simulink model "sistema_LTI_dinamica_residual"  (R2020b)
settings: Solver=VariableStepAuto  StartTime=0.0  StopTime=1.2  RelTol=1e-3
PreLoadFcn:
  | c4ModeloCompleto_var
PostLoadFcn:
  | c4ModeloCompleto_var
values from neighbouring files (symbols this model uses):
  Beq = bm+(bl)/r^2    (= 1.5e-05)    [c4ModeloCompleto_var.m]
  Jeq = Jm+(Jl/r^2)    (= 5.65099476805e-06)    [c4ModeloCompleto_var.m]
  lambda_m = 0.01546    [c4ModeloCompleto_var.m]
  Ld = 6.6e-3    (= 0.0066)    [c4ModeloCompleto_var.m]
  Lq = 5.8e-3    (= 0.0058)    [c4ModeloCompleto_var.m]
  Pp = 3    [c4ModeloCompleto_var.m]
  r = 314.3008    [c4ModeloCompleto_var.m]
undefined symbols (not defined in the file or in its folder): Rs, sigbuilder_block
settings Model: Creator=agustin  LastModifiedBy=agustin
settings DataIOCC: ReturnWorkspaceOutputs=off
settings DebuggingCC: ArithmeticOperatorsInVariantConditions=warning
settings SFSimCC: SimUseLocalCustomCode=off  CustomCodeUndefinedFunction=UseInterfaceOnly
settings RTWCC: RTWUseLocalCustomCode=off
settings CodeAppCC: StateflowObjectComments=on

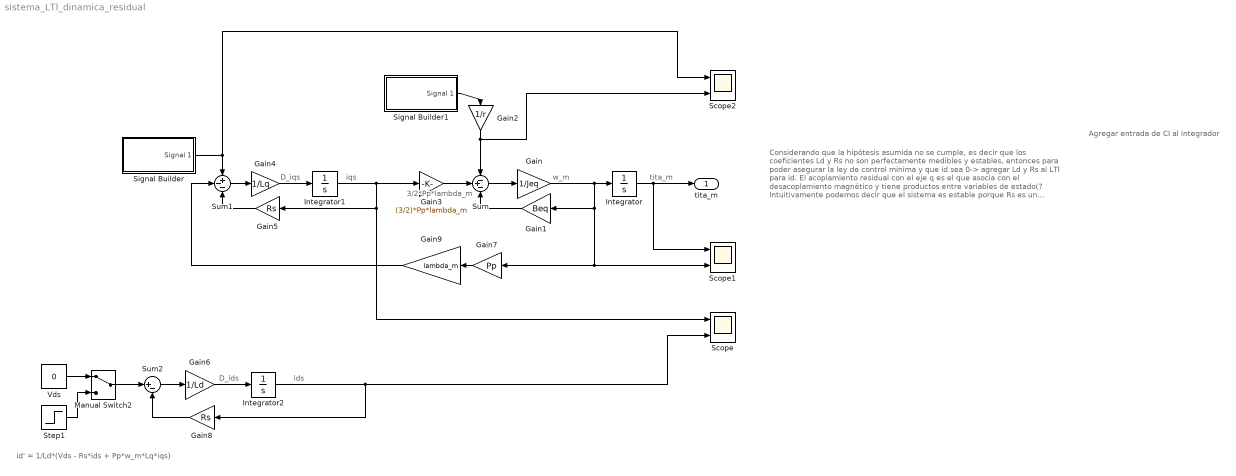
== system sistema_LTI_dinamica_residual ==
  note: id' = 1/Ld*(Vds - Rs*ids + Pp*w_m*Lq*iqs)
  note: 3/2*Pp*lambda_m
  note: Agregar entrada de CI al integrador
  note: Considerando que la hipótesis asumida no se cumple, es decir que los coeficientes Ld y Rs no son perfectamente medibles y estables, entonces para poder asegurar la ley de control mínima y que id sea 0-> agregar Ld y Rs al LTI para id.
      | El acoplamiento residual con el eje q es el que asocia con el desacoplamiento magnético y tiene productos entre variables de estado(?
      |
      | Intuitivamente podemos decir que el sistema es estable porque Rs es un término disipativo, este análisis se ve más en detalle al analizar polos.
      |
      | Se puede llegar a despreciar el acoplamiento NL porque el sistema es estable y se comporta como un filtro pasabajo con una constante de decaimiento Tau (Ld/Rs) que hace converger a la corriente a 0. El comportamiento como pasabajo se debe a que el sistema tiene un polo de primer orden
  note: tita_m
  note: w_m
  note: iqs
  note: D_iqs
  note: ids
  note: D_ids
  Gain : Gain  Gain=1/Jeq
  Gain1 : Gain  Gain=Beq
  Gain2 : Gain  Gain=1/r
  Gain3 : Gain  Gain=(3/2)*Pp*lambda_m
  Gain4 : Gain  Gain=1/Lq
  Gain5 : Gain  Gain=Rs
  Gain6 : Gain  Gain=1/Ld
  Gain7 : Gain  Gain=Pp
  Gain8 : Gain  Gain=Rs
  Gain9 : Gain  Gain=lambda_m
  Integrator : Integrator
  Integrator1 : Integrator
  Integrator2 : Integrator  InitialCondition=-.5
  Manual Switch2 : ManualSwitch
  Scope : Scope  NumInputPorts=2
  Scope1 : Scope  NumInputPorts=2
  Scope2 : Scope  NumInputPorts=2
  Signal Builder : Subsystem  Tag=STV Subsys  LoadFcn=sigbuilder_block('load');  StartFcn=sigbuilder_block('start');  StopFcn=sigbuilder_block('stop');  ClipboardFcn=sigbuilder_block('clipboard');  mask(Sigbuilder block){tuvar=[0:10]}
      mask help: Simulink:masks:SigbuilderBlock_MD
      mask init:
      | if ~strcmp(get_param(bdroot(gcbh),'SimulationStatus'),'stopped') tuvar = sigbuilder_block('maskInit'); end
      settings: CopyFcn=sigbuilder_block('copy');  DeleteFcn=sigbuilder_block('delete');  ModelCloseFcn=sigbuilder_block('modelClose');  PreSaveFcn=sigbuilder_block('preSave');  PauseFcn=sigbuilder_block('pause');  ContinueFcn=sigbuilder_block('continue');  NameChangeFcn=sigbuilder_block('namechange');  OpenFcn=sigbuilder_block('open',[437.25 154.5 550.5 357 ]);  CloseFcn=sigbuilder_block('close');
      mask Display: plot(0, 0, 100, 100,[2, 2, 32, 32, 2], [68, 8, 8, 68, 68],[32, 2], [38, 38], [32, 19, 2],[53, 60, 44], [32, 17, 17, 2],[16, 16, 31, 31]);txt = getActiveGroup(gcbh);text(2, 100, txt,'verticalAlignment', 'top');
  Signal Builder1 : Subsystem  Tag=STV Subsys  LoadFcn=sigbuilder_block('load');  StartFcn=sigbuilder_block('start');  StopFcn=sigbuilder_block('stop');  ClipboardFcn=sigbuilder_block('clipboard');  mask(Sigbuilder block){tuvar=[0:10]}
      mask help: Simulink:masks:SigbuilderBlock_MD
      mask init:
      | if ~strcmp(get_param(bdroot(gcbh),'SimulationStatus'),'stopped') tuvar = sigbuilder_block('maskInit'); end
      settings: CopyFcn=sigbuilder_block('copy');  DeleteFcn=sigbuilder_block('delete');  ModelCloseFcn=sigbuilder_block('modelClose');  PreSaveFcn=sigbuilder_block('preSave');  PauseFcn=sigbuilder_block('pause');  ContinueFcn=sigbuilder_block('continue');  NameChangeFcn=sigbuilder_block('namechange');  OpenFcn=sigbuilder_block('open',[0 0 1024.5 511.5 ]);  CloseFcn=sigbuilder_block('close');
      mask Display: plot(0, 0, 100, 100,[2, 2, 32, 32, 2], [68, 8, 8, 68, 68],[32, 2], [38, 38], [32, 19, 2],[53, 60, 44], [32, 17, 17, 2],[16, 16, 31, 31]);txt = getActiveGroup(gcbh);text(2, 100, txt,'verticalAlignment', 'top');
  Step1 : Step  SampleTime=0
  Sum : Sum  Inputs=-+-
  Sum1 : Sum  Inputs=+--
  Sum2 : Sum  Inputs=|+-
  "Vds " : Constant  Value=0
  tita_m : Outport  VectorParamsAs1DForOutWhenUnconnected=off
  wires:
  Sum/1 -> Gain/1
  Gain1/1 -> Sum/3
  Gain2/1 -> Sum/1, Scope2/2
  Gain3/1 -> Sum/2
  Gain4/1 -> Integrator1/1
  Sum1/1 -> Gain4/1
  Integrator1/1 -> Gain3/1, Gain5/1, Scope/1
  Gain5/1 -> Sum1/3
  Integrator/1 -> Scope1/1, tita_m/1
  Gain/1 -> Scope1/2, Gain7/1, Gain1/1, Integrator/1
  Gain6/1 -> Integrator2/1
  Sum2/1 -> Gain6/1
  Gain8/1 -> Sum2/2
  Gain9/1 -> Sum1/2
  Signal Builder/1(Signal 1) -> Scope2/1, Sum1/1
  Gain7/1 -> Gain9/1
  Signal Builder1/1(Signal 1) -> Gain2/1
  "Vds "/1 -> Manual Switch2/1
  Step1/1 -> Manual Switch2/2
  Manual Switch2/1 -> Sum2/1
  Integrator2/1 -> Scope/2, Gain8/1

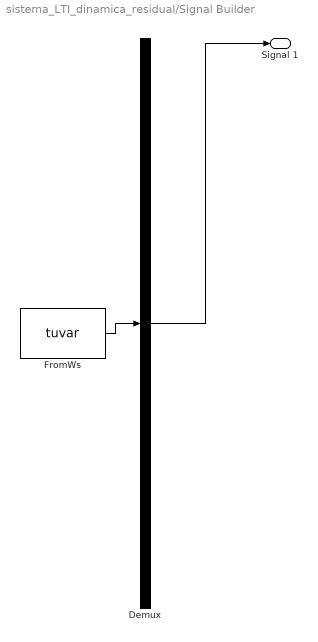
== system sistema_LTI_dinamica_residual/Signal Builder ==
  Demux : Demux  Tag=STV Demux  Outputs=1
      settings: DisplayOption=none
  FromWs : FromWorkspace  Tag=STV FromWs  VariableName=tuvar
      SigBuilderData=|
      | common.afterFinalStr = 'Extrapolate'
      | common.sampleTime = 0
      | dataSet.timeRange = [0 10]
      | dataSet.name = 'Group 1'
      | sbobj.Groups.Name = 'Group 1'
      | sbobj.Groups.Signals.Name = 'Signal 1'
      | sbobj.Groups.Signals.XData = [0 0.1 0.1 0.7 0.7 10]
      | sbobj.Groups.Signals.YData = [0 0 19.596 19.596 0 0]
  Signal 1 : Outport  Tag=STV Outport  VectorParamsAs1DForOutWhenUnconnected=off
  wires:
  Demux/1 -> Signal 1/1
  FromWs/1 -> Demux/1

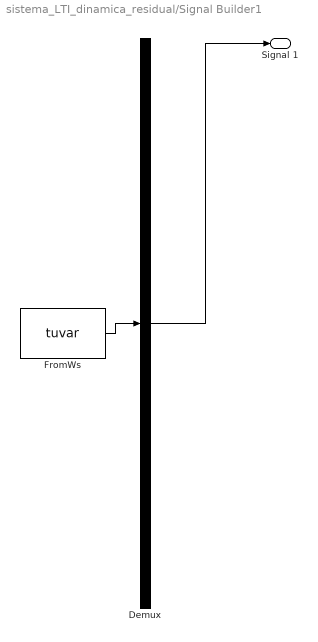
== system sistema_LTI_dinamica_residual/Signal Builder1 ==
  Demux : Demux  Tag=STV Demux  Outputs=1
      settings: DisplayOption=none
  FromWs : FromWorkspace  Tag=STV FromWs  VariableName=tuvar
      SigBuilderData=|
      | common.afterFinalStr = 'Extrapolate'
      | common.sampleTime = 0
      | dataSet.timeRange = [0 10]
      | dataSet.name = 'Group 1'
      | sbobj.Groups.Name = 'Group 1'
      | sbobj.Groups.Signals.Name = 'Signal 1'
      | sbobj.Groups.Signals.XData = [0 0.3 0.3 0.5 0.5 0.9 0.9 10]
      | sbobj.Groups.Signals.YData = [0 0 6.28 6.28 -6.28 -6.28 0 0]
  Signal 1 : Outport  Tag=STV Outport  VectorParamsAs1DForOutWhenUnconnected=off
  wires:
  Demux/1 -> Signal 1/1
  FromWs/1 -> Demux/1
